simulink model "IM_model"  (R2021a)
settings: Solver=FixedStepAuto  StartTime=0.0  StopTime=10  FixedStep=1e-5  RelTol=1e-3
InitFcn:
  | parameter
values from neighbouring files (symbols this model uses):
  f = 60    [parameter.m]
  Jm = 242.28    [parameter.m]
  L1a = X1a/2/pi/f    (= 6.73639212131e-05)    [parameter.m]
  L2a = X2a/2/pi/f    (= 6.41561024441e-05)    [parameter.m]
  Power = 4300e3    (= 4300000)    [parameter.m]
  pp = pole/2    (= 3)    [parameter.m]
  R1a = 2*R1    (= 0.001579662)    [parameter.m]
  R2a = 2*R2/0.933    (= 0.00113005359057)    [parameter.m]
  Rca = 2*Rc/0.9659    (= 45.9676985195)    [parameter.m]
  Vll = 700    [parameter.m]
libraries: spsACVoltageSourceLib x3, spsSeriesRLCBranchLib x3, spsRMSLib x3, spsCurrentMeasurementLib x2, spsGroundLib x1, spsAsynchronousMachineSIUnitsLib x1, spsMeanLib x1, eePowerMeasurement x1, spsThreePhaseVIMeasurementLib x1, spspowerguiLib x1, spsVoltageMeasurementLib x1
settings Model: Creator=enes_  LastModifiedBy=enes_

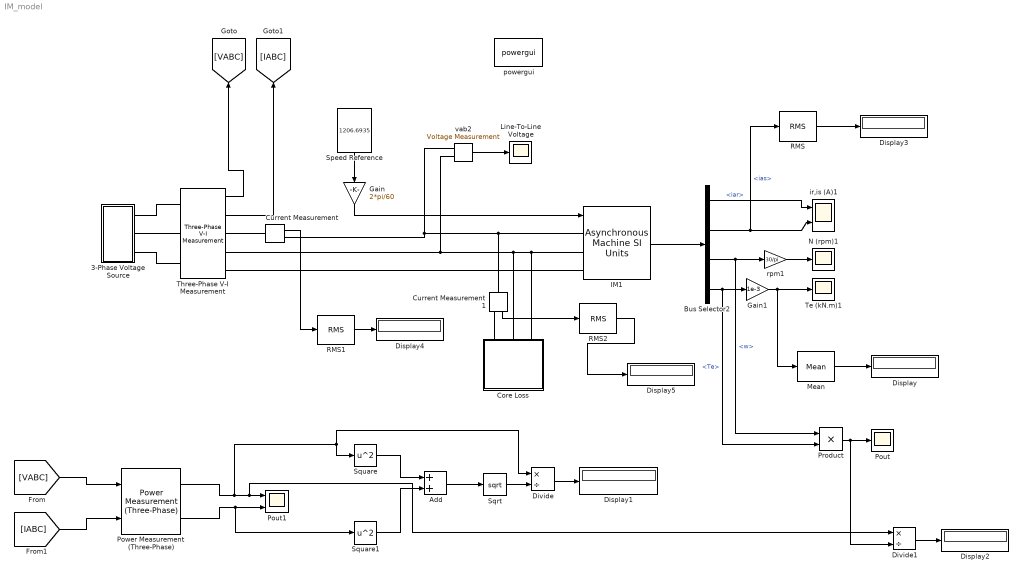
== system IM_model ==
  3-Phase Voltage Source : Subsystem
  Add : Sum
  Bus Selector2 : BusSelector  OutputSignals=iar,ias,w,Te
  Core Loss : Subsystem
  Current Measurement : spsCurrentMeasurementLib/Current Measurement  PhasorSimulation=off  OutputType=Complex  PSBequivalent=0
  Current Measurement1 : spsCurrentMeasurementLib/Current Measurement  PhasorSimulation=off  OutputType=Complex  PSBequivalent=0
  Display{,1..5} (6 alike) : Display
  Divide : Product  Inputs=*/
  Divide1 : Product  Inputs=*/
  Gain : Gain  Gain=2*pi/60
  Gain1 : Gain  Gain=1e-3
  IM1 : spsAsynchronousMachineSIUnitsLib/Asynchronous Machine SI Units  RotorType=Squirrel-cage  PresetModel=No  MechanicalLoad=Speed w  ShowDetailedParameters=on  ReferenceFrame=Stationary  Units=SI  MeasurementBus=on  NominalParameters=[Power/2 Vll f]  VoltageRatio=1  Stator=[R1a L1a]  Rotor=[R2a L2a]  Cage1=[ 0.022 0.226/377]  Cage2=[ 0.022 0.226/377]  Lm=Lma  Mechanical=[Jm 0 pp]  PolePairs=pp  InitialConditions="[ 1,0   0,0,0   0,0,0 ]"  SimulateSaturation=off  Saturation=[14.03593122, 27.81365428, 53.79336849, 72.68890987, 97.98006896, 148.6815601, 215.7428561, 302.9841135, 428.7778367 ; 230, 322, 414, 460, 506, 552, 598, 644, 690]  LoadFlowParameters=0  TsPowergui=0  TsBlock=-1  IterativeModel=Trapezoidal non iterative  IterativeDiscreteModel=Trapezoidal non iterative  Pmec=0
      settings: AttributesFormatString=\n
  Line-To-Line Voltage : Scope
  Mean : spsMeanLib/Mean  Freq=60  Vinit=0  Ts=0
  N (rpm)1 : Scope
  Pout : Scope
  Pout1 : Scope  NumInputPorts=2
  Power Measurement (Three-Phase) : eePowerMeasurement/Power Measurement (Three-Phase)  LabelModeActiveChoice=Continuous  F=60  K=[1]  Seq=Positive  Ts=0
      settings: SourceProductBaseCode=PS
  Product : Product
  RMS : spsRMSLib/RMS  TrueRMS=off  Freq=60  RMSInit=0  Ts=0
  RMS1 : spsRMSLib/RMS  TrueRMS=off  Freq=60  RMSInit=0  Ts=0
  RMS2 : spsRMSLib/RMS  TrueRMS=off  Freq=60  RMSInit=0  Ts=0
  Speed Reference : Constant  Value=1206.6935
  Sqrt : Sqrt  SaturateOnIntegerOverflow=on
  Square : Math  Operator=square  SaturateOnIntegerOverflow=on
  Square1 : Math  Operator=square  SaturateOnIntegerOverflow=on
  Te (kN.m)1 : Scope
  Three-Phase V-I Measurement : spsThreePhaseVIMeasurementLib/Three-Phase V-I Measurement  VoltageMeasurement=phase-to-ground  SetLabelV=off  LabelV=Vabc  Vpu=off  VpuLL=off  CurrentMeasurement=yes  SetLabelI=off  LabelI=Iabc  Ipu=off  Pbase=100e6  Vbase=500e3  OutputType=Complex  PhasorSimulation=off  PSBequivalent=0
  ir,is (A)1 : Scope  NumInputPorts=2
  powergui : spspowerguiLib/powergui  SimulationMode=Continuous  SampleTime=0  frequency=60  Iterations=50  frequencyindice=60  Pbase=100e6  ErrMax=1e-4  UnitsV=kV  UnitsW=MW  buscounter=0  FunctionMessages=off  echomessages=off  EnableUseOfTLC=off  CurrentSourceSwitches=off  DisableSnubberDevices=off  DisableRonSwitches=off  DisableVfSwitches=off  DisplayEquations=off  AutomaticDiscreteSolvers=off  SolverType=Tustin  Interpol=off  ExternalGateDelay=off  methode=off  Ts=0  x0status=blocks  SPID=on  SwTol=0  HookPort=off  NonlinearTolerance=1e-4  nMaxIteration=100  ContinueOnMaxIteration=off  RestoreLinks=warning  ResistiveCurrentMeasurement=off  Frange=[0:2:500]  Ylog=off  Xlog=on  ShowGrid=off  save=off  variable=ZData  structure=0  ZoomFFT=on  StartTime=0.0  cycles=1  DisplayStyle=1  fundamental=60  FreqAxis=off  MaxFrequency=1000  frequencyindicesteady=1  RmsSteady=1  display=off
  rpm1 : Gain  Gain=30/pi  SaturateOnIntegerOverflow=on  OutDataTypeStr=Inherit: Same as input  ParamDataTypeStr=Inherit: Same as input
  vab2 : spsVoltageMeasurementLib/Voltage Measurement  Tag=PoWeRsYsTeMmEaSuReMeNt  PhasorSimulation=off  OutputType=Magnitude  PSBequivalent=0
  wires:
  Gain1/1 -> Mean/1, Te (kN.m)1/1
  Bus Selector2/2 -> RMS/1, ir,is (A)1/2  "<ias>"
  rpm1/1 -> N (rpm)1/1
  vab2/1 -> Line-To-Line Voltage/1
  Bus Selector2/1 -> ir,is (A)1/1  "<iar>"
  Bus Selector2/4 -> Product/2, Gain1/1  "<Te>"
  IM1/1 -> Bus Selector2/1
  Bus Selector2/3 -> Product/1, rpm1/1  "<w>"
  Gain/1 -> IM1/1
  Speed Reference/1 -> Gain/1
  Mean/1 -> Display/1
  Product/1 -> Divide1/2, Pout/1
  Three-Phase V-I Measurement/1 -> [VABC]
  Three-Phase V-I Measurement/2 -> [IABC]
  [VABC] -> Power Measurement (Three-Phase)/1
  [IABC] -> Power Measurement (Three-Phase)/2
  Power Measurement (Three-Phase)/1 -> Divide/1, Square/1, Divide1/1, Pout1/1
  Power Measurement (Three-Phase)/2 -> Square1/1, Pout1/2
  Square/1 -> Add/1
  Square1/1 -> Add/2
  Add/1 -> Sqrt/1
  Sqrt/1 -> Divide/2
  Divide/1 -> Display1/1
  Divide1/1 -> Display2/1
  RMS/1 -> Display3/1
  RMS1/1 -> Display4/1
  Current Measurement/1 -> RMS1/1
  Current Measurement1/1 -> RMS2/1
  RMS2/1 -> Display5/1
  connections:
  vab2/LConn2 -- IM1/LConn2 -- Core Loss/LConn3 -- Core Loss/LConn2 -- Three-Phase V-I Measurement/RConn2
  vab2/LConn1 -- Current Measurement/RConn1 -- Current Measurement1/LConn1 -- IM1/LConn1
  Three-Phase V-I Measurement/LConn1 -- 3-Phase Voltage Source/RConn1
  Three-Phase V-I Measurement/LConn3 -- 3-Phase Voltage Source/RConn3
  Three-Phase V-I Measurement/LConn2 -- 3-Phase Voltage Source/RConn2
  Three-Phase V-I Measurement/RConn3 -- IM1/LConn3
  Current Measurement/LConn1 -- Three-Phase V-I Measurement/RConn1
  Current Measurement1/RConn1 -- Core Loss/LConn1

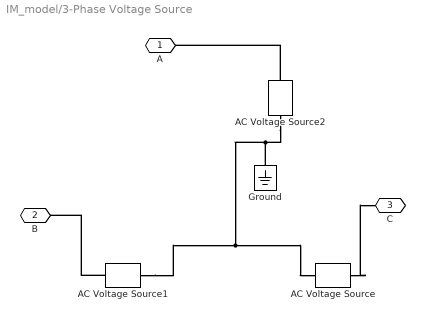
== system IM_model/3-Phase Voltage Source ==
  AC Voltage Source : spsACVoltageSourceLib/AC Voltage Source  Amplitude=Vll/sqrt(3)*sqrt(2)  Phase=120  Frequency=f  SampleTime=0  Measurements=None  BusType=swing  Pref=10e3  Qref=0  Qmin=-inf  Qmax=+inf
  AC Voltage Source1 : spsACVoltageSourceLib/AC Voltage Source  Amplitude=Vll/sqrt(3)*sqrt(2)  Phase=240  Frequency=f  SampleTime=0  Measurements=None  BusType=swing  Pref=10e3  Qref=0  Qmin=-inf  Qmax=+inf
  AC Voltage Source2 : spsACVoltageSourceLib/AC Voltage Source  Amplitude=Vll/sqrt(3)*sqrt(2)  Phase=0  Frequency=f  SampleTime=0  Measurements=None  BusType=swing  Pref=10e3  Qref=0  Qmin=-inf  Qmax=+inf
  Ground : spsGroundLib/Ground  LConnTagsString=a
  A : PMIOPort  Side=Right
  B : PMIOPort  Port=2  Side=Right
  C : PMIOPort  Port=3  Side=Right
  connections:
  AC Voltage Source2/LConn1 -- AC Voltage Source1/LConn1 -- AC Voltage Source/LConn1 -- Ground/LConn1
  AC Voltage Source1/RConn1 -- B/RConn1
  AC Voltage Source2/RConn1 -- A/RConn1
  AC Voltage Source/RConn1 -- C/RConn1

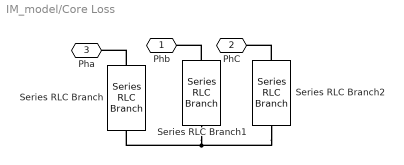
== system IM_model/Core Loss ==
  Series RLC Branch : spsSeriesRLCBranchLib/Series RLC Branch  LConnTagsString=__new0  RConnTagsString=__new0  BranchType=R  Resistance=Rca  Inductance=1e-3  SetiL0=off  InitialCurrent=0  Capacitance=1e-6  Setx0=off  InitialVoltage=0  Measurements=None
  Series RLC Branch1 : spsSeriesRLCBranchLib/Series RLC Branch  LConnTagsString=__new0  RConnTagsString=__new0  BranchType=R  Resistance=Rca  Inductance=1e-3  SetiL0=off  InitialCurrent=0  Capacitance=1e-6  Setx0=off  InitialVoltage=0  Measurements=None
  Series RLC Branch2 : spsSeriesRLCBranchLib/Series RLC Branch  LConnTagsString=__new0  RConnTagsString=__new0  BranchType=R  Resistance=Rca  Inductance=1e-3  SetiL0=off  InitialCurrent=0  Capacitance=1e-6  Setx0=off  InitialVoltage=0  Measurements=None
  Phb : PMIOPort  Side=Left
  PhC : PMIOPort  Port=2  Side=Left
  Pha : PMIOPort  Port=3  Side=Left
  connections:
  Series RLC Branch2/RConn1 -- Series RLC Branch1/RConn1 -- Series RLC Branch/RConn1
  Series RLC Branch/LConn1 -- Pha/RConn1
  Series RLC Branch1/LConn1 -- Phb/RConn1
  Series RLC Branch2/LConn1 -- PhC/RConn1
